simulink model "dcmotorbasiconline"  (R2022a)
settings: Solver=VariableStepAuto  StartTime=0.0  StopTime=10.0  RelTol=1e-3
model workspace (MAT data in the model file):
  K = 0.01
  L = 0.5
  b = 0.1
  ke = 0.01
  r = 1
libraries: nesl_utility x1
settings Model: Creator=DELL  LastModifiedBy=DELL

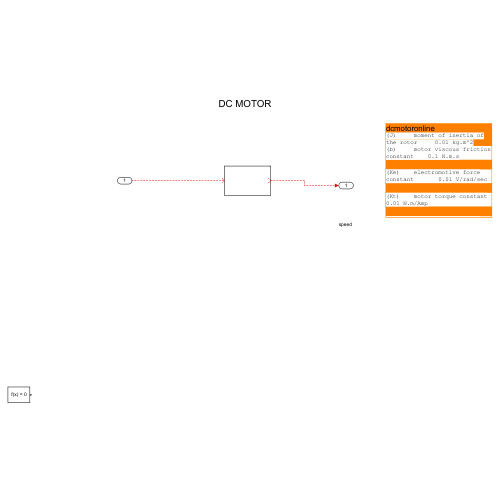
[thumbnail: Simulink's stored preview of the top-level diagram]
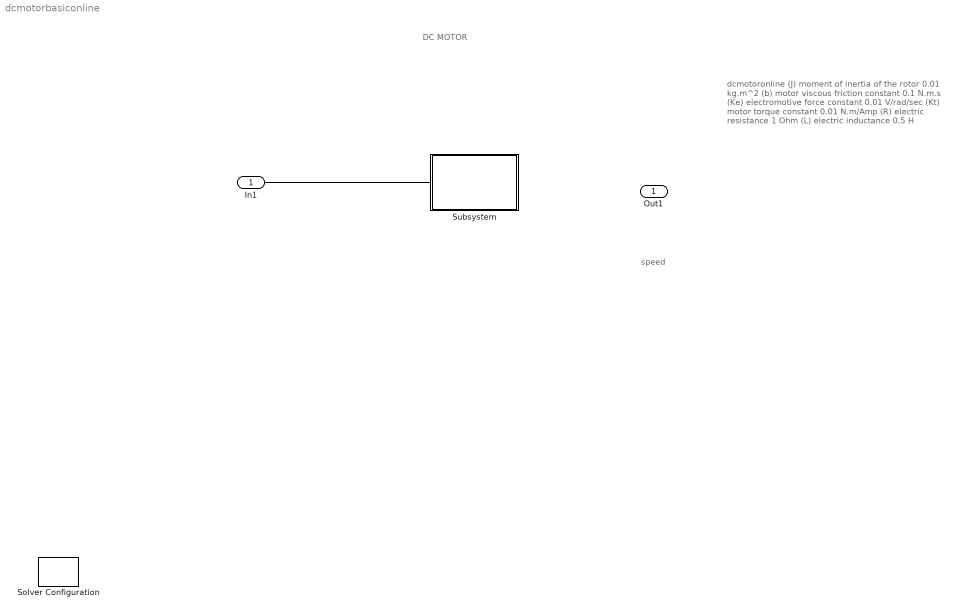
== system dcmotorbasiconline ==
  note: dcmotoronline
      | (J) moment of inertia of the rotor 0.01 kg.m^2
      | (b) motor viscous friction constant 0.1 N.m.s
      | (Ke) electromotive force constant 0.01 V/rad/sec
      | (Kt) motor torque constant 0.01 N.m/Amp
      | (R) electric resistance 1 Ohm
      | (L) electric inductance 0.5 H
  note: speed
  note: DC MOTOR
  In1 : Inport
  Solver Configuration : nesl_utility/Solver Configuration  PhysicalDomain=network_engine_domain  SubClassName=solver  LeftPortType=input  RightPortType=generic  Tones=[]  Harmonics=[]  SimulateNoise=off  Profile=off  UseLocalSampling=off  EnableSwitchedLinearOptims=on  FrequencyDomain=off  UseCCode=off  RelTol=0.001  AbsTol=0.001  MinStep=1e-09  ToWorkspace=off  RevertToSquareIcSolve=off  NumHomotopyIterations=100  PhasorMode=off  PhasorModeNumHarmonics=1  IndexReductionMethod=DerivativeReplacement  DoDC=off  ResidualTolerance=1e-09  UseLocalSolver=off  LocalSolverChoice=NE_BACKWARD_EULER_ADVANCER  LocalSolverSampleTime=0.001  DoFixedCost=off  MaxNonlinIter=3  MaxModeIter=2  ComputeImpulses=off  ImpulseIterations=2  LinearAlgebra=auto  LinearAlgebraNumThread=0  EquationFormulation=NE_TIME_EF  DelaysMemoryBudget=1024  AutomaticFiltering=on  FilteringTimeConstant=0.001  PartitionStorageMethod=AS_NEEDED  PartitionMemoryBudget=1024  PartitionMethod=ROBUST
      settings: SourceProductBaseCode=SS,PW,VE
  Subsystem : Subsystem
  Out1 : Outport
  wires:
  In1/1 -> ?
  ? -> Out1/1

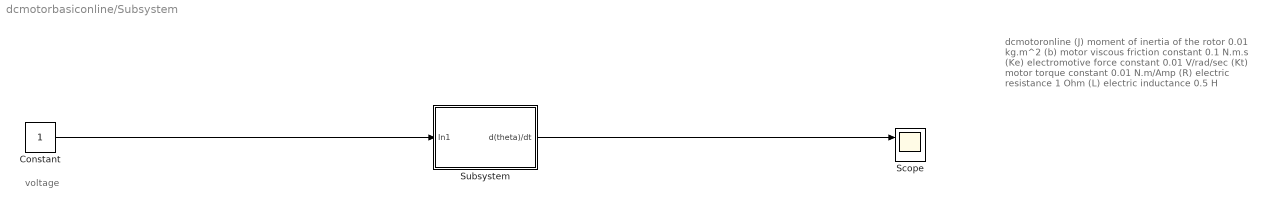
== system dcmotorbasiconline/Subsystem ==
  note: voltage
  note: dcmotoronline
      | (J) moment of inertia of the rotor 0.01 kg.m^2
      | (b) motor viscous friction constant 0.1 N.m.s
      | (Ke) electromotive force constant 0.01 V/rad/sec
      | (Kt) motor torque constant 0.01 N.m/Amp
      | (R) electric resistance 1 Ohm
      | (L) electric inductance 0.5 H
  Constant : Constant
  Scope : Scope  NumInputPorts=2
  Subsystem : Subsystem
  wires:
  Constant/1 -> Subsystem/1(In1)
  Subsystem/1(d(theta)/dt) -> Scope/1

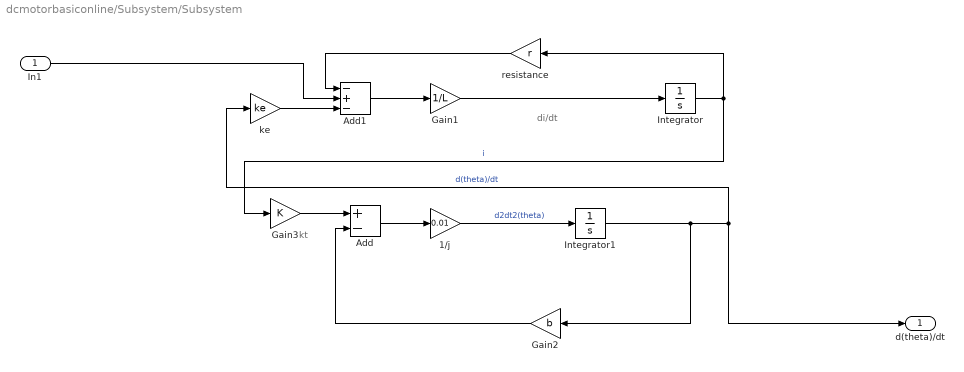
== system dcmotorbasiconline/Subsystem/Subsystem ==
  note: kt
  note: di/dt
  In1 : Inport
  1/j : Gain  Gain=0.01
  Add : Sum  Inputs=+-
  Add1 : Sum  Inputs=-+-
  Gain1 : Gain  Gain=1/L
  Gain2 : Gain  Gain=b
  Gain3 : Gain  Gain=K
  Integrator : Integrator
  Integrator1 : Integrator
  ke : Gain  Gain=ke
  resistance : Gain  Gain=r
  d(theta)/dt : Outport
  wires:
  1/j/1 -> Integrator1/1  "d2dt2(theta)"
  Integrator/1 -> Gain3/1, resistance/1  "i"
  Integrator1/1 -> Gain2/1, ke/1, d(theta)/dt/1  "d(theta)/dt"
  ke/1 -> Add1/3
  Gain2/1 -> Add/2
  Gain1/1 -> Integrator/1
  Add/1 -> 1/j/1
  Add1/1 -> Gain1/1
  resistance/1 -> Add1/1
  Gain3/1 -> Add/1
  In1/1 -> Add1/2
